simulink model "HANcoder_Olimexino"  (R2015a)
settings: Solver=FixedStepDiscrete  SolverMode=SingleTasking  StartTime=0.0  StopTime=2  FixedStep=0.01  RelTol=1e-3
PreLoadFcn:
  | librarySetup
  | eval([bdroot,'_startup']) %Calling [modelName]_startup.m
undefined symbols (not defined in the file or in its folder): CON4, D13, HANtuneOverride, LED1
libraries: HANcoder_STM32_Target x9, simulink x2
CloseFcn:
  | rtwprivate ssgencode ModelCloseRequest mytest
settings Model: CovSFcnEnable=off  Creator=Jason van Kolfschoten  LastModifiedBy=TestServer
settings SolverCC: PositivePriorityOrder=on
settings DataIOCC: SignalLoggingSaveFormat=ModelDataLogs  SaveOutput=off  SaveTime=off
settings OptimizationCC: BlockReduction=off  InlineParams=on  DefaultUnderspecifiedDataType=single  InlineInvariantSignals=on  ExpressionDepthLimit=2147483647  StateBitsets=on  DataBitsets=on  ZeroExternalMemoryAtStartup=off  ZeroInternalMemoryAtStartup=off  InitFltsAndDblsToZero=on  NoFixptDivByZeroProtection=on  EfficientFloat2IntCast=on  OptimizeModelRefInitCode=on
settings DebuggingCC: SaveWithDisabledLinksMsg=none  SaveWithParameterizedLinksMsg=none  CheckSSInitialOutputMsg=off  UnderspecifiedInitializationDetection=Classic  MergeDetectMultiDrivingBlocksExec=none  SignalResolutionControl=TryResolveAll  SolverPrmCheckMsg=warning  InheritedTsInSrcMsg=none  MultiTaskDSMMsg=warning  MultiTaskCondExecSysMsg=none  ParameterPrecisionLossMsg=none  FcnCallInpInsideContextMsg=EnableAllAsWarning  StateNameClashWarn=warning
settings HardwareCC: ProdLargestAtomicInteger=Long  ProdLargestAtomicFloat=Double  ProdIntDivRoundTo=Zero  ProdEndianess=LittleEndian  ProdHWDeviceType=ARM Compatible->ARM Cortex  TargetEndianess=LittleEndian  TargetHWDeviceType=Infineon->TriCore
settings RTWCC: SystemTargetFile=ert.tlc  MakeCommand=make_rtw SHELL= HANcoder_PORTABLE=1 HANcoder_BOOTLOADER=0  TemplateMakefile=Olimexino_STM32_gcc.tmf  Description=Real-Time Workshop Embedded Coder (no auto configuration)
settings CodeAppCC: ForceParamTrailComments=on  IgnoreCustomStorageClasses=off  SimulinkDataObjDesc=on  CustomSymbolStrGlobalVar=rt$N$M  CustomSymbolStrType=$N$M  CustomSymbolStrFcn=$N$M$F  CustomSymbolStrMacro=$N$M  InsertBlockDesc=on  InternalIdentifier=Classic
settings ERTTargetCC: TargetFcnLib=ansi_tfl_tmw.mat  GenerateSampleERTMain=off  ParMdlRefBuildCompliant=on  CompOptLevelCompliant=on  ConcurrentExecutionCompliant=on  IncludeMdlTerminateFcn=off  SuppressErrorStatus=on  ERTFirstTimeCompliant=on  SupportNonFinite=off  SupportContinuousTime=off  SupportVariableSizeSignals=off  ModelStepFunctionPrototypeControlCompliant=on  CPPClassGenCompliant=on  GenerateASAP2=on  ERTCustomFileTemplate=example_file_process.tlc
settings ConfigComp: Description=Design Verifier Custom Configuration Component  DVMaxProcessTime=600  DVDisplayUnsatisfiableObjectives=on  DVAutomaticStubbing=off  DVSubSystemToStub=7.76600366011452e-316  DVParameterNames=7.76600366011452e-316  DVParameterConstraints=7.76600366011452e-316  DVParameterUseInAnalysis=7.76600366011452e-316  DVModelCoverageObjectives=MCDC  DVMaxTestCaseSteps=500  DVTestSuiteOptimization=CombinedObjectives  DVDetectActiveLogic=on  DVDetectFloatOverflow=off  DVSaveHarnessModel=on

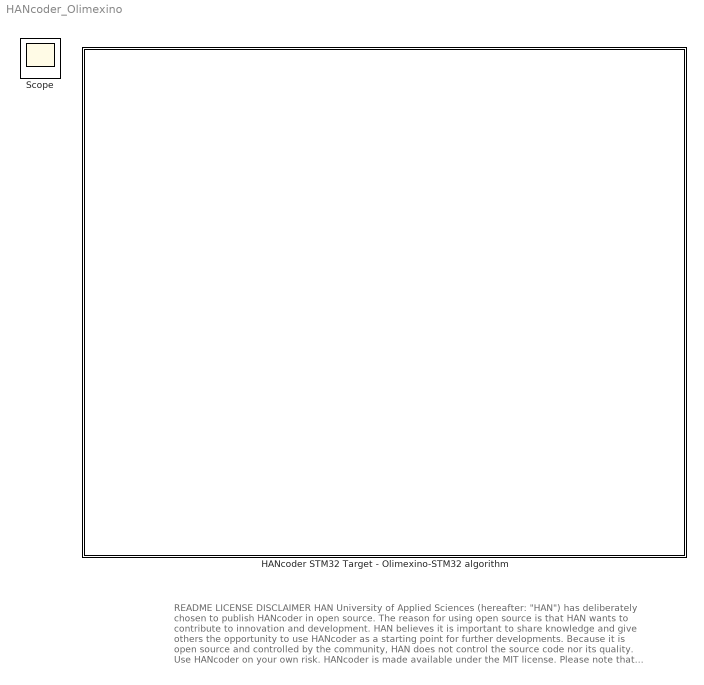
== system HANcoder_Olimexino ==
  note: README
      |
      | LICENSE
      |
      | DISCLAIMER
      |
      | HAN University of Applied Sciences (hereafter: "HAN") has deliberately chosen
      | to publish HANcoder in open source. The reason for using open source is that
      | HAN wants to contribute to innovation and development. HAN believes it is
      | important to share knowledge and give others the opportunity to use HANcoder
      | as a starting point for further developments. Because it is open source and
      | controlled by the community, HAN does not control the source code nor its
      | quality. Use HANcoder on your own risk. HANcoder is made available under the
      | MIT license. Please note that this license contains an exclusion of liability.
  HANcoder STM32 Target - Olimexino-STM32 algorithm : Subsystem  mask(TopLevelSubsystem){}
      mask Display: image(imread('Olimexino_STM32_HAN.jpg'))
  Scope : Scope
      settings: TimeRange=10  LimitDataPoints=on  MaxDataPoints=7500  SaveToWorkspace=off  SaveName=ScopeData  YMin=-1  YMax=1  SampleTime=-1  DataFormat=Array

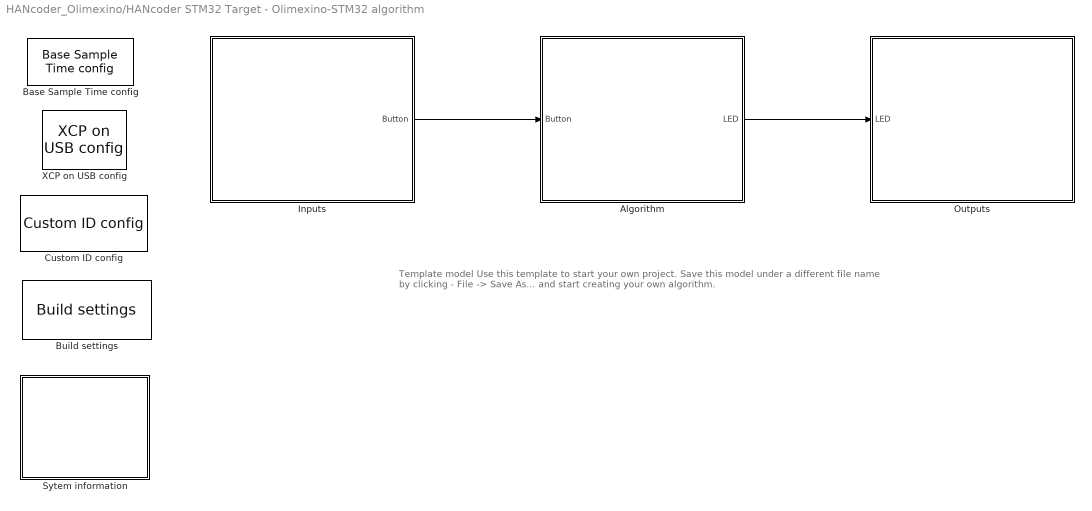
== system HANcoder_Olimexino/HANcoder STM32 Target - Olimexino-STM32 algorithm ==
  note: Template model
      | Use this template to start your own project. Save this model
      | under a different file name by clicking - File -> Save As... and
      | start creating your own algorithm.
  Algorithm : Subsystem
  Base Sample Time config : HANcoder_STM32_Target/Olimexino STM32/System Config/Base Sample Time config  Tag=HANcoder_TARGET_STM32_Olimexino  Description=HANcoder Target STM32-Olimexino blockset version 1.1  baseSampleTime=10  extraStack=25
  Build settings : HANcoder_STM32_Target/Olimexino STM32/System Config/Build settings  Tag=HANcoder_TARGET_STM32_Olimexino  AutoASAP2add=on  AutoFlash=off
  Custom ID config : HANcoder_STM32_Target/Olimexino STM32/System Config/Custom ID config  Tag=HANcoder_TARGET_STM32_Olimexino  softID=softwareID  softNUM=1
  Inputs : Subsystem
  Outputs : Subsystem
  Sytem information : Subsystem
  XCP on USB config : HANcoder_STM32_Target/Olimexino STM32/System Config/XCP on USB config  Tag=HANcoder_TARGET_STM32_Olimexino
  wires:
  Inputs/1(Button) -> Algorithm/1(Button)
  Algorithm/1(LED) -> Outputs/1(LED)

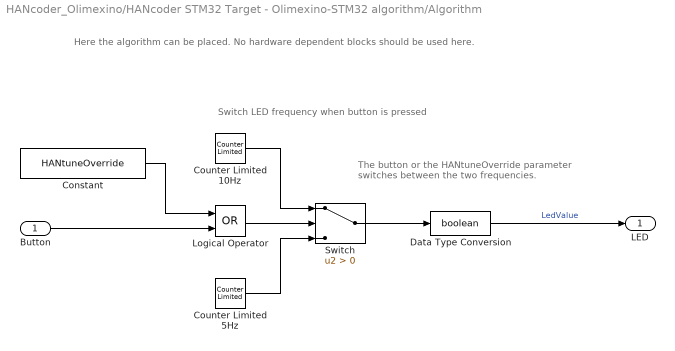
== system HANcoder_Olimexino/HANcoder STM32 Target - Olimexino-STM32 algorithm/Algorithm ==
  note: The button or the HANtuneOverride parameter
      | switches between the two frequencies.
  note: Switch LED frequency when button is pressed
  note: Here the algorithm can be placed. No hardware dependent blocks should be used here.
  Button : Inport
  Constant : Constant  Value=HANtuneOverride  OutDataTypeStr=boolean
  Counter Limited 10Hz : simulink/Sources/Counter Limited  uplimit=1  tsamp=0.1
  Counter Limited 5Hz : simulink/Sources/Counter Limited  uplimit=1  tsamp=0.2
  Data Type Conversion : DataTypeConversion  OutDataTypeStr=boolean
  Logical Operator : Logic  Operator=OR  AllPortsSameDT=off  OutDataTypeStr=boolean
  Switch : Switch  Criteria=u2 > Threshold
  LED : Outport
  wires:
  Data Type Conversion/1 -> LED/1  "LedValue"
  Counter Limited 5Hz/1 -> Switch/3
  Switch/1 -> Data Type Conversion/1
  Button/1 -> Logical Operator/2
  Logical Operator/1 -> Switch/2
  Constant/1 -> Logical Operator/1
  Counter Limited 10Hz/1 -> Switch/1

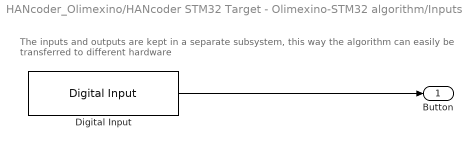
== system HANcoder_Olimexino/HANcoder STM32 Target - Olimexino-STM32 algorithm/Inputs ==
  note: The inputs and outputs are kept in a separate subsystem, this way the algorithm can easily be transferred to different hardware
  Digital Input : HANcoder_STM32_Target/Olimexino STM32/Digital Inputs/Digital Input  Tag=HANcoder_TARGET_STM32_Olimexino  pinID=Pushbutton - BUT/BOOT0 - 5V Tolerant  config=Pulldown  tsamp=-1
  Button : Outport
  wires:
  Digital Input/1 -> Button/1

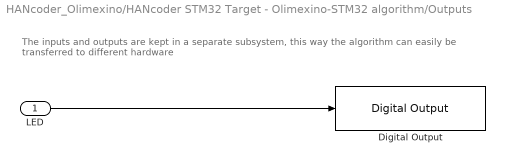
== system HANcoder_Olimexino/HANcoder STM32 Target - Olimexino-STM32 algorithm/Outputs ==
  note: The inputs and outputs are kept in a separate subsystem, this way the algorithm can easily be transferred to different hardware
  LED : Inport
  Digital Output : HANcoder_STM32_Target/Olimexino STM32/Digital Outputs/Digital Output  Tag=HANcoder_TARGET_STM32_Olimexino  pinID=CON4 - D13/LED1  config=Push pull  tsamp=-1
  wires:
  LED/1 -> Digital Output/1

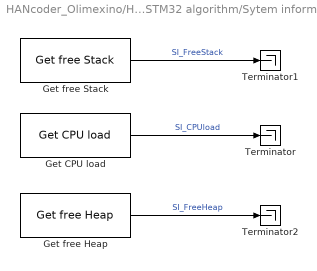
== system HANcoder_Olimexino/HANcoder STM32 Target - Olimexino-STM32 algorithm/Sytem information ==
  Get CPU load : HANcoder_STM32_Target/Olimexino STM32/System Management/Get CPU load  Tag=HANcoder_TARGET_STM32_Olimexino  mode=Current CPU load  tsamp=-1
  Get free Heap : HANcoder_STM32_Target/Olimexino STM32/System Management/Get free Heap  Tag=HANcoder_TARGET_STM32_Olimexino  tsamp=-1
  Get free Stack : HANcoder_STM32_Target/Olimexino STM32/System Management/Get free Stack  Tag=HANcoder_TARGET_STM32_Olimexino  taskIdx=Application Control Task  tsamp=-1
  Terminator : Terminator
  Terminator1 : Terminator
  Terminator2 : Terminator
  wires:
  Get CPU load/1 -> Terminator/1  "SI_CPUload"
  Get free Stack/1 -> Terminator1/1  "SI_FreeStack"
  Get free Heap/1 -> Terminator2/1  "SI_FreeHeap"
